simulink model "inverted_pendulum_sim_fuz_dk_view"  (R2021a)
settings: Solver=VariableStepAuto  StartTime=0.0  StopTime=10  RelTol=1e-3
values from neighbouring files (symbols this model uses):
  g = 9.8    [inverted_pendulum_fuz.m]
  kd0 = 0.005    [inverted_pendulum_fuz.m]
  ki0 = 0    [inverted_pendulum_fuz.m]
  kp0 = 0.116    [inverted_pendulum_fuz.m]
  L = 0.12    [inverted_pendulum_fuz.m]
  m = 0.017    [inverted_pendulum_fuz.m]
  M = 0.07    [inverted_pendulum_fuz.m]
  Mm = 20*0.001    (= 0.02)    [inverted_pendulum_fuz.m]
  R = 0.065    [inverted_pendulum_fuz.m]
  Rm = 26.3/2*0.01    (= 0.1315)    [inverted_pendulum_fuz.m]
  theta1_ini = pi*(20)/180    (= 0.349065850399)    [inverted_pendulum_fuz.m]
libraries: fuzblock x2
settings Model: Creator=18214  LastModifiedBy=18214

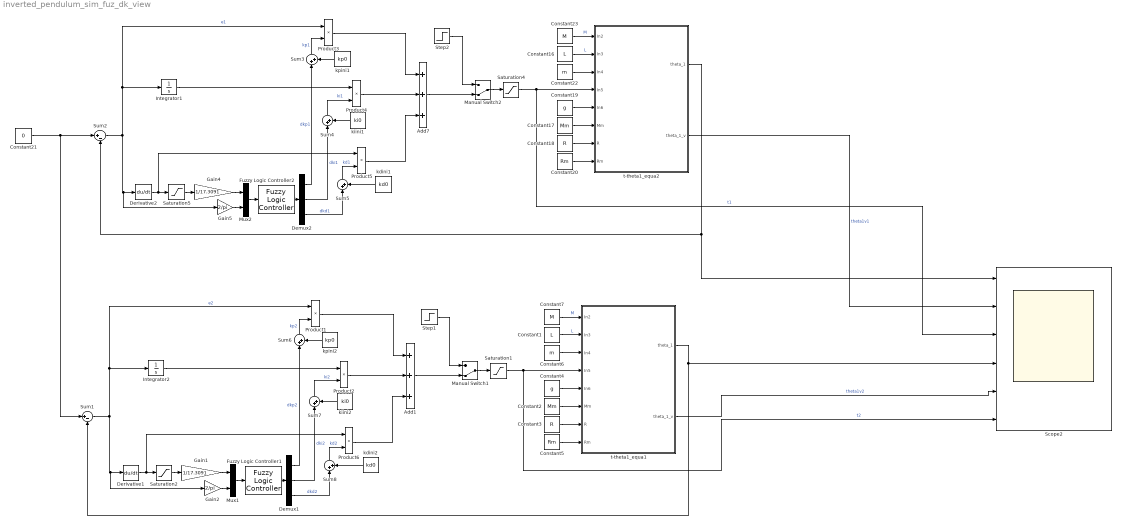
== system inverted_pendulum_sim_fuz_dk_view ==
  Add1 : Sum  Inputs=+++
  Add7 : Sum  Inputs=+++
  Constant1 : Constant  Value=L
  Constant16 : Constant  Value=L
  Constant17 : Constant  Value=Mm
  Constant18 : Constant  Value=R
  Constant19 : Constant  Value=g
  Constant2 : Constant  Value=Mm
  Constant20 : Constant  Value=Rm
  Constant21 : Constant  Value=0
  Constant22 : Constant  Value=m
  Constant23 : Constant  Value=M
  Constant3 : Constant  Value=R
  Constant4 : Constant  Value=g
  Constant5 : Constant  Value=Rm
  Constant6 : Constant  Value=m
  Constant7 : Constant  Value=M
  Demux1 : Demux  Outputs=3
  Demux2 : Demux  Outputs=3
  Derivative1 : Derivative
  Derivative2 : Derivative
  Fuzzy Logic Controller1 : fuzblock/Fuzzy Logic  Controller  FIS='fuzzyctr_dk13.fis'  OutputSampleNumber=101  DataType=double  FuzzifiedInputs=off  RuleFiringStrengths=off  RuleOutputs=off  AggregatedOutputs=off  SimulateUsing=Interpreted execution  OutOfRangeInputValueMessage=warning  NoRuleFiredMessage=warning  EmptyOutputFuzzySetMessage=warning
  Fuzzy Logic Controller2 : fuzblock/Fuzzy Logic  Controller  FIS='fuzzyctr_dk10.fis'  OutputSampleNumber=101  DataType=double  FuzzifiedInputs=off  RuleFiringStrengths=off  RuleOutputs=off  AggregatedOutputs=off  SimulateUsing=Interpreted execution  OutOfRangeInputValueMessage=warning  NoRuleFiredMessage=warning  EmptyOutputFuzzySetMessage=warning
  Gain1 : Gain  Gain=1/17.3091
  Gain2 : Gain  Gain=2/pi
  Gain4 : Gain  Gain=1/17.3091
  Gain5 : Gain  Gain=2/pi
  Integrator1 : Integrator
  Integrator2 : Integrator
  Manual Switch1 : ManualSwitch  CurrentSetting=0
  Manual Switch2 : ManualSwitch  CurrentSetting=0
  Mux1 : Mux  Inputs=2
  Mux2 : Mux  Inputs=2
  Product{1..6} (6 alike) : Product
  Saturation1 : Saturate  UpperLimit=inf  LowerLimit=-inf
  Saturation2 : Saturate  UpperLimit=17.3091  LowerLimit=-17.3091
  Saturation4 : Saturate  UpperLimit=inf  LowerLimit=-inf
  Saturation5 : Saturate  UpperLimit=17.3091  LowerLimit=-17.3091
  Scope2 : Scope  NumInputPorts=6
  Step1 : Step  After=0  SampleTime=0
  Step2 : Step  After=0  SampleTime=0
  Sum1 : Sum  Inputs=|+-
  Sum2 : Sum  Inputs=|+-
  Sum{3..8} (6 alike) : Sum  Inputs=|++
  kdini1 : Constant  Value=kd0
  kdini2 : Constant  Value=kd0
  kiini1 : Constant  Value=ki0
  kiini2 : Constant  Value=ki0
  kpini1 : Constant  Value=kp0
  kpini2 : Constant  Value=kp0
  t-theta1_equa1 : Subsystem
  t-theta1_equa2 : Subsystem
  wires:
  Constant17/1 -> t-theta1_equa2/6(Mm)
  Product5/1 -> Add7/3
  Constant22/1 -> t-theta1_equa2/3(In4)
  Constant18/1 -> t-theta1_equa2/7(R)
  Demux2/3 -> Sum5/1  "dkd1"
  Saturation5/1 -> Gain4/1
  t-theta1_equa2/2(theta_1_v) -> Scope2/2  "theta1v1"
  Saturation4/1 -> t-theta1_equa2/4(In5), Scope2/3  "t1"
  Product4/1 -> Add7/2
  Manual Switch2/1 -> Saturation4/1
  Demux2/1 -> Sum3/1  "dkp1"
  Sum2/1 -> Product3/1, Integrator1/1, Gain5/1, Derivative2/1  "e1"
  Add7/1 -> Manual Switch2/2
  Product3/1 -> Add7/1
  Constant19/1 -> t-theta1_equa2/5(In6)
  Gain4/1 -> Mux2/1
  Gain5/1 -> Mux2/2
  kiini1/1 -> Sum4/2
  Fuzzy Logic Controller2/1 -> Demux2/1
  Mux2/1 -> Fuzzy Logic Controller2/1
  Integrator1/1 -> Product4/1
  Constant16/1 -> t-theta1_equa2/2(In3)  "L"
  Step2/1 -> Manual Switch2/1
  Constant20/1 -> t-theta1_equa2/8(Rm)
  Sum5/1 -> Product5/2  "kd1"
  t-theta1_equa2/1(theta_1) -> Scope2/1, Sum2/2
  Derivative2/1 -> Product5/1, Saturation5/1
  kdini1/1 -> Sum5/2
  kpini1/1 -> Sum3/2
  Sum4/1 -> Product4/2  "ki1"
  Constant23/1 -> t-theta1_equa2/1(In2)  "M"
  Demux2/2 -> Sum4/1  "dki1"
  Sum3/1 -> Product3/2  "kp1"
  Integrator2/1 -> Product2/1
  Gain1/1 -> Mux1/1
  Constant7/1 -> t-theta1_equa1/1(In2)  "M"
  Sum7/1 -> Product2/2  "ki2"
  Step1/1 -> Manual Switch1/1
  Constant5/1 -> t-theta1_equa1/8(Rm)
  Constant6/1 -> t-theta1_equa1/3(In4)
  kpini2/1 -> Sum6/2
  Manual Switch1/1 -> Saturation1/1
  Derivative1/1 -> Product6/1, Saturation2/1
  Demux1/3 -> Sum8/1  "dkd2"
  Product1/1 -> Add1/1
  t-theta1_equa1/1(theta_1) -> Sum1/2, Scope2/4
  Add1/1 -> Manual Switch1/2
  Sum1/1 -> Product1/1, Integrator2/1, Gain2/1, Derivative1/1  "e2"
  Product6/1 -> Add1/3
  Fuzzy Logic Controller1/1 -> Demux1/1
  Constant4/1 -> t-theta1_equa1/5(In6)
  Mux1/1 -> Fuzzy Logic Controller1/1
  kiini2/1 -> Sum7/2
  Demux1/2 -> Sum7/1  "dki2"
  Gain2/1 -> Mux1/2
  Product2/1 -> Add1/2
  Demux1/1 -> Sum6/1  "dkp2"
  Sum8/1 -> Product6/2  "kd2"
  Constant2/1 -> t-theta1_equa1/6(Mm)
  Sum6/1 -> Product1/2  "kp2"
  Saturation1/1 -> Scope2/6, t-theta1_equa1/4(In5)  "t2"
  kdini2/1 -> Sum8/2
  t-theta1_equa1/2(theta_1_v) -> Scope2/5  "theta1v2"
  Constant3/1 -> t-theta1_equa1/7(R)
  Constant1/1 -> t-theta1_equa1/2(In3)  "L"
  Saturation2/1 -> Gain1/1
  Constant21/1 -> Sum1/1, Sum2/1

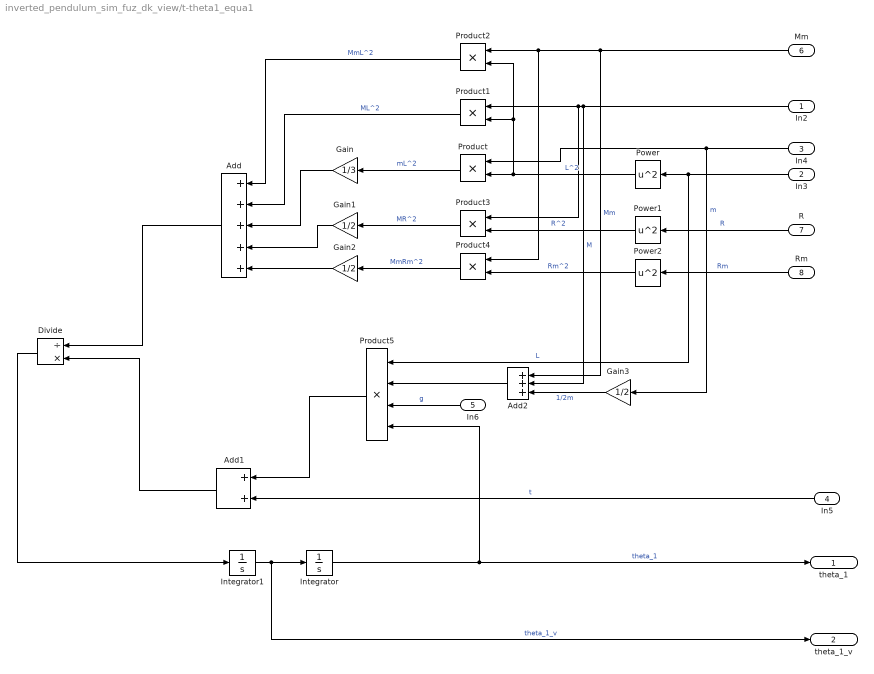
== system inverted_pendulum_sim_fuz_dk_view/t-theta1_equa1 ==
  In2 : Inport
  In3 : Inport  Port=2
  In4 : Inport  Port=3
  In5 : Inport  Port=4
  In6 : Inport  Port=5
  Mm : Inport  Port=6
  R : Inport  Port=7
  Rm : Inport  Port=8
  Add : Sum  Inputs=+++++
  Add1 : Sum
  Add2 : Sum  Inputs=+++
  Divide : Product  Inputs=/*
  Gain : Gain  Gain=1/3
  Gain1 : Gain  Gain=1/2
  Gain2 : Gain  Gain=1/2
  Gain3 : Gain  Gain=1/2
  Integrator : Integrator  InitialCondition=theta1_ini  LowerSaturationLimit=-pi
  Integrator1 : Integrator
  Power : Math  Operator=square  SaturateOnIntegerOverflow=on
  Power1 : Math  Operator=square  SaturateOnIntegerOverflow=on
  Power2 : Math  Operator=square  SaturateOnIntegerOverflow=on
  Product{,1..4} (5 alike) : Product
  Product5 : Product  Inputs=4
  theta_1 : Outport
  theta_1_v : Outport  Port=2
  wires:
  Integrator/1 -> Product5/4, theta_1/1  "theta_1"
  Integrator1/1 -> theta_1_v/1, Integrator/1  "theta_1_v"
  Mm/1 -> Product4/1, Product2/1, Add2/1  "Mm"
  R/1 -> Power1/1  "R"
  Rm/1 -> Power2/1  "Rm"
  In3/1 -> Product5/1, Power/1  "L"
  Power/1 -> Product2/2, Product1/2, Product/2  "L^2"
  In4/1 -> Product/1, Gain3/1  "m"
  Product/1 -> Gain/1  "mL^2"
  In2/1 -> Product1/1, Product3/1, Add2/2  "M"
  Product1/1 -> Add/2  "ML^2"
  Product2/1 -> Add/1  "MmL^2"
  Power1/1 -> Product3/2  "R^2"
  Power2/1 -> Product4/2  "Rm^2"
  Product3/1 -> Gain1/1  "MR^2"
  Product4/1 -> Gain2/1  "MmRm^2"
  Gain2/1 -> Add/5
  Gain1/1 -> Add/4
  Gain/1 -> Add/3
  Add/1 -> Divide/1
  Add1/1 -> Divide/2
  In5/1 -> Add1/2  "t"
  Gain3/1 -> Add2/3  "1/2m"
  Add2/1 -> Product5/2
  In6/1 -> Product5/3  "g"
  Divide/1 -> Integrator1/1
  Product5/1 -> Add1/1

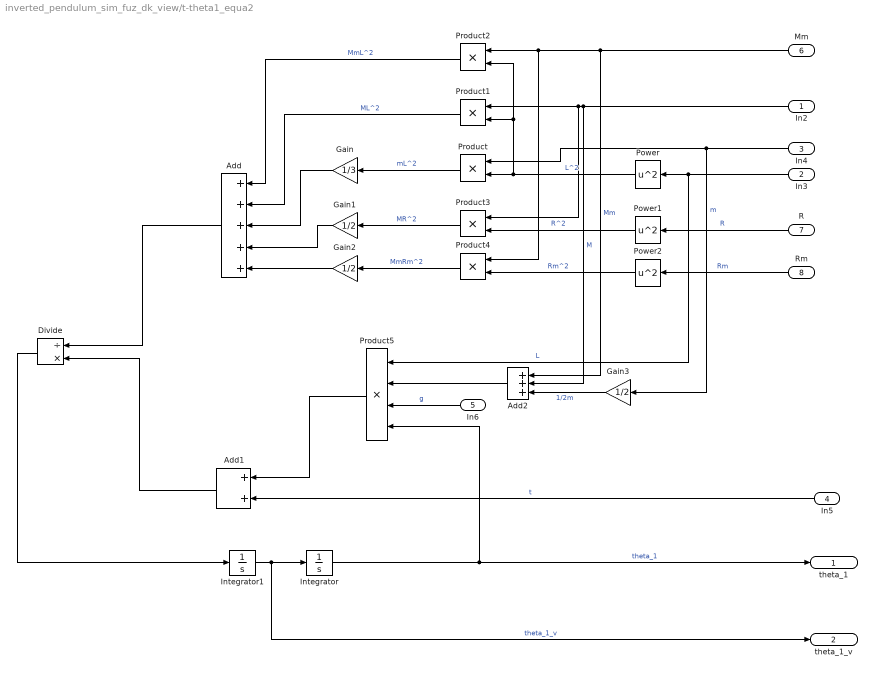
== system inverted_pendulum_sim_fuz_dk_view/t-theta1_equa2 ==
  In2 : Inport
  In3 : Inport  Port=2
  In4 : Inport  Port=3
  In5 : Inport  Port=4
  In6 : Inport  Port=5
  Mm : Inport  Port=6
  R : Inport  Port=7
  Rm : Inport  Port=8
  Add : Sum  Inputs=+++++
  Add1 : Sum
  Add2 : Sum  Inputs=+++
  Divide : Product  Inputs=/*
  Gain : Gain  Gain=1/3
  Gain1 : Gain  Gain=1/2
  Gain2 : Gain  Gain=1/2
  Gain3 : Gain  Gain=1/2
  Integrator : Integrator  InitialCondition=theta1_ini  LowerSaturationLimit=-pi
  Integrator1 : Integrator
  Power : Math  Operator=square  SaturateOnIntegerOverflow=on
  Power1 : Math  Operator=square  SaturateOnIntegerOverflow=on
  Power2 : Math  Operator=square  SaturateOnIntegerOverflow=on
  Product{,1..4} (5 alike) : Product
  Product5 : Product  Inputs=4
  theta_1 : Outport
  theta_1_v : Outport  Port=2
  wires:
  Integrator/1 -> Product5/4, theta_1/1  "theta_1"
  Integrator1/1 -> theta_1_v/1, Integrator/1  "theta_1_v"
  Mm/1 -> Product4/1, Product2/1, Add2/1  "Mm"
  R/1 -> Power1/1  "R"
  Rm/1 -> Power2/1  "Rm"
  In3/1 -> Product5/1, Power/1  "L"
  Power/1 -> Product2/2, Product1/2, Product/2  "L^2"
  In4/1 -> Product/1, Gain3/1  "m"
  Product/1 -> Gain/1  "mL^2"
  In2/1 -> Product1/1, Product3/1, Add2/2  "M"
  Product1/1 -> Add/2  "ML^2"
  Product2/1 -> Add/1  "MmL^2"
  Power1/1 -> Product3/2  "R^2"
  Power2/1 -> Product4/2  "Rm^2"
  Product3/1 -> Gain1/1  "MR^2"
  Product4/1 -> Gain2/1  "MmRm^2"
  Gain2/1 -> Add/5
  Gain1/1 -> Add/4
  Gain/1 -> Add/3
  Add/1 -> Divide/1
  Add1/1 -> Divide/2
  In5/1 -> Add1/2  "t"
  Gain3/1 -> Add2/3  "1/2m"
  Add2/1 -> Product5/2
  In6/1 -> Product5/3  "g"
  Divide/1 -> Integrator1/1
  Product5/1 -> Add1/1
